simulink model "TST_MeUn_VD"  (R2016b)
settings: Solver=FixedStepDiscrete  StartTime=0.0  StopTime=simTime  FixedStep=sampleTime  RelTol=1e-3
values from neighbouring files (symbols this model uses):
  testCase = 1    [initTST_MeUn_VD_001.m]
libraries: simulink x9, UnitTest_Lib x7
settings Model: Creator=zhengjinyan  LastModifiedBy=zhengjinyan
settings DebuggingCC: SignalRangeChecking=error

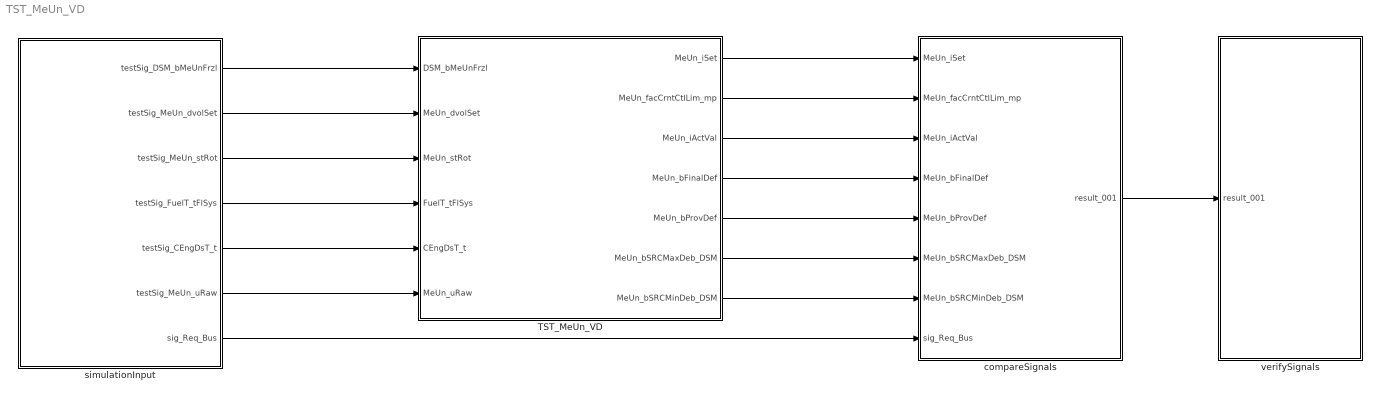
== system TST_MeUn_VD ==
  TST_MeUn_VD : Subsystem
  compareSignals : Subsystem
  simulationInput : Subsystem
  verifySignals : Subsystem
  wires:
  simulationInput/1(testSig_DSM_bMeUnFrzl) -> TST_MeUn_VD/1(DSM_bMeUnFrzl)
  simulationInput/2(testSig_MeUn_dvolSet) -> TST_MeUn_VD/2(MeUn_dvolSet)
  simulationInput/3(testSig_MeUn_stRot) -> TST_MeUn_VD/3(MeUn_stRot)
  simulationInput/4(testSig_FuelT_tFlSys) -> TST_MeUn_VD/4(FuelT_tFlSys)
  simulationInput/5(testSig_CEngDsT_t) -> TST_MeUn_VD/5(CEngDsT_t)
  simulationInput/6(testSig_MeUn_uRaw) -> TST_MeUn_VD/6(MeUn_uRaw)
  TST_MeUn_VD/1(MeUn_iSet) -> compareSignals/1(MeUn_iSet)
  TST_MeUn_VD/2(MeUn_facCrntCtlLim_mp) -> compareSignals/2(MeUn_facCrntCtlLim_mp)
  TST_MeUn_VD/3(MeUn_iActVal) -> compareSignals/3(MeUn_iActVal)
  TST_MeUn_VD/4(MeUn_bFinalDef) -> compareSignals/4(MeUn_bFinalDef)
  TST_MeUn_VD/5(MeUn_bProvDef) -> compareSignals/5(MeUn_bProvDef)
  TST_MeUn_VD/6(MeUn_bSRCMaxDeb_DSM) -> compareSignals/6(MeUn_bSRCMaxDeb_DSM)
  TST_MeUn_VD/7(MeUn_bSRCMinDeb_DSM) -> compareSignals/7(MeUn_bSRCMinDeb_DSM)
  simulationInput/7(sig_Req_Bus) -> compareSignals/8(sig_Req_Bus)
  compareSignals/1(result_001) -> verifySignals/1(result_001)

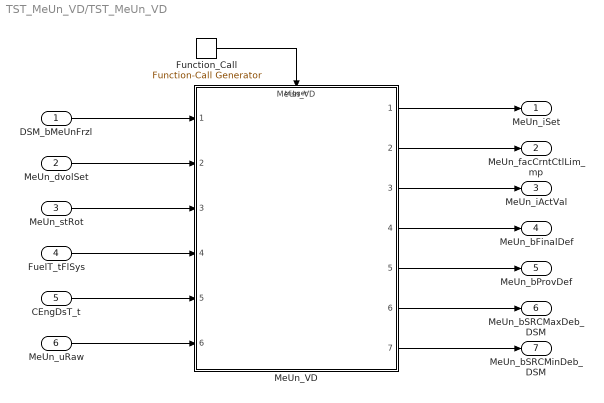
== system TST_MeUn_VD/TST_MeUn_VD ==
  DSM_bMeUnFrzl : Inport
  MeUn_dvolSet : Inport  Port=2
  MeUn_stRot : Inport  Port=3
  FuelT_tFlSys : Inport  Port=4
  CEngDsT_t : Inport  Port=5
  MeUn_uRaw : Inport  Port=6
  Function_Call : simulink/Ports & Subsystems/Function-Call Generator  sample_time=sampleTime  numberOfIterations=1
  MeUn_VD : ModelReference  ModelNameDialog=MeUn_VD  SimulationMode=Normal  ModelReferenceVersion=1.27  TriggerPortName=function  TriggerPortTriggerType=function-call  TriggerPortStatesWhenEnabling=held
  MeUn_iSet : Outport
  MeUn_facCrntCtlLim_mp : Outport  Port=2
  MeUn_iActVal : Outport  Port=3
  MeUn_bFinalDef : Outport  Port=4
  MeUn_bProvDef : Outport  Port=5
  MeUn_bSRCMaxDeb_DSM : Outport  Port=6
  MeUn_bSRCMinDeb_DSM : Outport  Port=7
  wires:
  Function_Call/1 -> MeUn_VD/Trigger
  DSM_bMeUnFrzl/1 -> MeUn_VD/1
  MeUn_dvolSet/1 -> MeUn_VD/2
  MeUn_stRot/1 -> MeUn_VD/3
  FuelT_tFlSys/1 -> MeUn_VD/4
  CEngDsT_t/1 -> MeUn_VD/5
  MeUn_uRaw/1 -> MeUn_VD/6
  MeUn_VD/1 -> MeUn_iSet/1
  MeUn_VD/2 -> MeUn_facCrntCtlLim_mp/1
  MeUn_VD/3 -> MeUn_iActVal/1
  MeUn_VD/4 -> MeUn_bFinalDef/1
  MeUn_VD/5 -> MeUn_bProvDef/1
  MeUn_VD/6 -> MeUn_bSRCMaxDeb_DSM/1
  MeUn_VD/7 -> MeUn_bSRCMinDeb_DSM/1

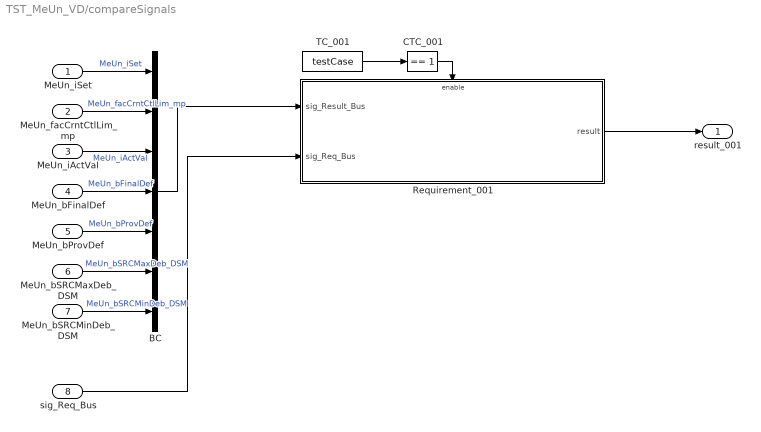
== system TST_MeUn_VD/compareSignals ==
  MeUn_iSet : Inport
  MeUn_facCrntCtlLim_mp : Inport  Port=2
  MeUn_iActVal : Inport  Port=3
  MeUn_bFinalDef : Inport  Port=4
  MeUn_bProvDef : Inport  Port=5
  MeUn_bSRCMaxDeb_DSM : Inport  Port=6
  MeUn_bSRCMinDeb_DSM : Inport  Port=7
  sig_Req_Bus : Inport  Port=8
  BC : BusCreator  Inputs=7
  CTC_001 : simulink/Logic and Bit Operations/Compare To Constant  relop===  const=1  OutDataTypeStr=boolean
  Requirement_001 : Subsystem
  TC_001 : Constant  Value=testCase
  result_001 : Outport
  wires:
  MeUn_iSet/1 -> BC/1  "MeUn_iSet"
  MeUn_facCrntCtlLim_mp/1 -> BC/2  "MeUn_facCrntCtlLim_mp"
  MeUn_iActVal/1 -> BC/3  "MeUn_iActVal"
  MeUn_bFinalDef/1 -> BC/4  "MeUn_bFinalDef"
  MeUn_bProvDef/1 -> BC/5  "MeUn_bProvDef"
  MeUn_bSRCMaxDeb_DSM/1 -> BC/6  "MeUn_bSRCMaxDeb_DSM"
  MeUn_bSRCMinDeb_DSM/1 -> BC/7  "MeUn_bSRCMinDeb_DSM"
  TC_001/1 -> CTC_001/1
  CTC_001/1 -> Requirement_001/Enable
  sig_Req_Bus/1 -> Requirement_001/2(sig_Req_Bus)
  BC/1 -> Requirement_001/1(sig_Result_Bus)
  Requirement_001/1(result) -> result_001/1

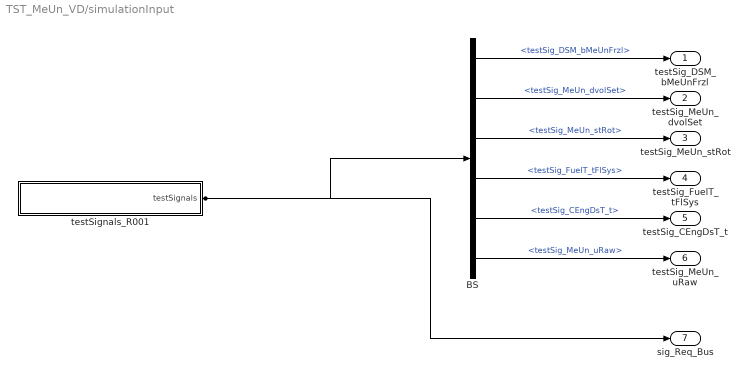
== system TST_MeUn_VD/simulationInput ==
  BS : BusSelector  OutputSignals=testSig_DSM_bMeUnFrzl,testSig_MeUn_dvolSet,testSig_MeUn_stRot,testSig_FuelT_tFlSys,testSig_CEngDsT_t,testSig_MeUn_uRaw
  testSignals_R001 : Subsystem
  testSig_DSM_bMeUnFrzl : Outport
  testSig_MeUn_dvolSet : Outport  Port=2
  testSig_MeUn_stRot : Outport  Port=3
  testSig_FuelT_tFlSys : Outport  Port=4
  testSig_CEngDsT_t : Outport  Port=5
  testSig_MeUn_uRaw : Outport  Port=6
  sig_Req_Bus : Outport  Port=7
  wires:
  BS/1 -> testSig_DSM_bMeUnFrzl/1  "<testSig_DSM_bMeUnFrzl>"
  BS/2 -> testSig_MeUn_dvolSet/1  "<testSig_MeUn_dvolSet>"
  BS/3 -> testSig_MeUn_stRot/1  "<testSig_MeUn_stRot>"
  BS/4 -> testSig_FuelT_tFlSys/1  "<testSig_FuelT_tFlSys>"
  BS/5 -> testSig_CEngDsT_t/1  "<testSig_CEngDsT_t>"
  BS/6 -> testSig_MeUn_uRaw/1  "<testSig_MeUn_uRaw>"
  testSignals_R001/1(testSignals) -> BS/1, sig_Req_Bus/1

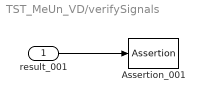
== system TST_MeUn_VD/verifySignals ==
  result_001 : Inport
  Assertion_001 : Assertion  Enabled=off
  wires:
  result_001/1 -> Assertion_001/1

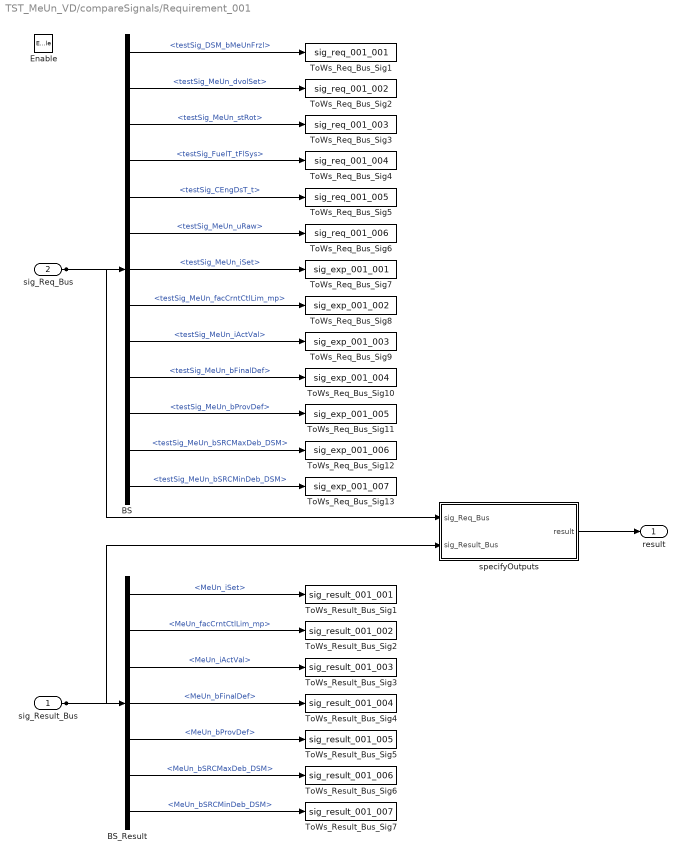
== system TST_MeUn_VD/compareSignals/Requirement_001 ==
  sig_Result_Bus : Inport
  sig_Req_Bus : Inport  Port=2
  Enable : EnablePort
  BS : BusSelector  OutputSignals=testSig_DSM_bMeUnFrzl,testSig_MeUn_dvolSet,testSig_MeUn_stRot,testSig_FuelT_tFlSys,testSig_CEngDsT_t,testSig_MeUn_uRaw,testSig_MeUn_iSet,testSig_MeUn_facCrntCtlLim_mp,testSig_MeUn_iActVal,testSig_MeUn_bFinalDef,testSig_MeUn_bProvDef,testSig_MeUn_bSRCMaxDeb_DSM,testSig_MeUn_bSRCMinDeb_DSM
  BS_Result : BusSelector  OutputSignals=MeUn_iSet,MeUn_facCrntCtlLim_mp,MeUn_iActVal,MeUn_bFinalDef,MeUn_bProvDef,MeUn_bSRCMaxDeb_DSM,MeUn_bSRCMinDeb_DSM
  ToWs_Req_Bus_Sig1 : ToWorkspace  VariableName=sig_req_001_001  SaveFormat=Structure With Time
  ToWs_Req_Bus_Sig10 : ToWorkspace  VariableName=sig_exp_001_004  SaveFormat=Structure With Time
  ToWs_Req_Bus_Sig11 : ToWorkspace  VariableName=sig_exp_001_005  SaveFormat=Structure With Time
  ToWs_Req_Bus_Sig12 : ToWorkspace  VariableName=sig_exp_001_006  SaveFormat=Structure With Time
  ToWs_Req_Bus_Sig13 : ToWorkspace  VariableName=sig_exp_001_007  SaveFormat=Structure With Time
  ToWs_Req_Bus_Sig2 : ToWorkspace  VariableName=sig_req_001_002  SaveFormat=Structure With Time
  ToWs_Req_Bus_Sig3 : ToWorkspace  VariableName=sig_req_001_003  SaveFormat=Structure With Time
  ToWs_Req_Bus_Sig4 : ToWorkspace  VariableName=sig_req_001_004  SaveFormat=Structure With Time
  ToWs_Req_Bus_Sig5 : ToWorkspace  VariableName=sig_req_001_005  SaveFormat=Structure With Time
  ToWs_Req_Bus_Sig6 : ToWorkspace  VariableName=sig_req_001_006  SaveFormat=Structure With Time
  ToWs_Req_Bus_Sig7 : ToWorkspace  VariableName=sig_exp_001_001  SaveFormat=Structure With Time
  ToWs_Req_Bus_Sig8 : ToWorkspace  VariableName=sig_exp_001_002  SaveFormat=Structure With Time
  ToWs_Req_Bus_Sig9 : ToWorkspace  VariableName=sig_exp_001_003  SaveFormat=Structure With Time
  ToWs_Result_Bus_Sig1 : ToWorkspace  VariableName=sig_result_001_001  SaveFormat=Structure With Time
  ToWs_Result_Bus_Sig2 : ToWorkspace  VariableName=sig_result_001_002  SaveFormat=Structure With Time
  ToWs_Result_Bus_Sig3 : ToWorkspace  VariableName=sig_result_001_003  SaveFormat=Structure With Time
  ToWs_Result_Bus_Sig4 : ToWorkspace  VariableName=sig_result_001_004  SaveFormat=Structure With Time
  ToWs_Result_Bus_Sig5 : ToWorkspace  VariableName=sig_result_001_005  SaveFormat=Structure With Time
  ToWs_Result_Bus_Sig6 : ToWorkspace  VariableName=sig_result_001_006  SaveFormat=Structure With Time
  ToWs_Result_Bus_Sig7 : ToWorkspace  VariableName=sig_result_001_007  SaveFormat=Structure With Time
  specifyOutputs : Subsystem
  result : Outport
  wires:
  sig_Req_Bus/1 -> BS/1, specifyOutputs/1(sig_Req_Bus)
  BS/1 -> ToWs_Req_Bus_Sig1/1  "<testSig_DSM_bMeUnFrzl>"
  BS/2 -> ToWs_Req_Bus_Sig2/1  "<testSig_MeUn_dvolSet>"
  BS/3 -> ToWs_Req_Bus_Sig3/1  "<testSig_MeUn_stRot>"
  BS/4 -> ToWs_Req_Bus_Sig4/1  "<testSig_FuelT_tFlSys>"
  BS/5 -> ToWs_Req_Bus_Sig5/1  "<testSig_CEngDsT_t>"
  BS/6 -> ToWs_Req_Bus_Sig6/1  "<testSig_MeUn_uRaw>"
  BS/7 -> ToWs_Req_Bus_Sig7/1  "<testSig_MeUn_iSet>"
  BS/8 -> ToWs_Req_Bus_Sig8/1  "<testSig_MeUn_facCrntCtlLim_mp>"
  BS/9 -> ToWs_Req_Bus_Sig9/1  "<testSig_MeUn_iActVal>"
  BS/10 -> ToWs_Req_Bus_Sig10/1  "<testSig_MeUn_bFinalDef>"
  BS/11 -> ToWs_Req_Bus_Sig11/1  "<testSig_MeUn_bProvDef>"
  BS/12 -> ToWs_Req_Bus_Sig12/1  "<testSig_MeUn_bSRCMaxDeb_DSM>"
  BS/13 -> ToWs_Req_Bus_Sig13/1  "<testSig_MeUn_bSRCMinDeb_DSM>"
  sig_Result_Bus/1 -> BS_Result/1, specifyOutputs/2(sig_Result_Bus)
  BS_Result/1 -> ToWs_Result_Bus_Sig1/1  "<MeUn_iSet>"
  BS_Result/2 -> ToWs_Result_Bus_Sig2/1  "<MeUn_facCrntCtlLim_mp>"
  BS_Result/3 -> ToWs_Result_Bus_Sig3/1  "<MeUn_iActVal>"
  BS_Result/4 -> ToWs_Result_Bus_Sig4/1  "<MeUn_bFinalDef>"
  BS_Result/5 -> ToWs_Result_Bus_Sig5/1  "<MeUn_bProvDef>"
  BS_Result/6 -> ToWs_Result_Bus_Sig6/1  "<MeUn_bSRCMaxDeb_DSM>"
  BS_Result/7 -> ToWs_Result_Bus_Sig7/1  "<MeUn_bSRCMinDeb_DSM>"
  specifyOutputs/1(result) -> result/1

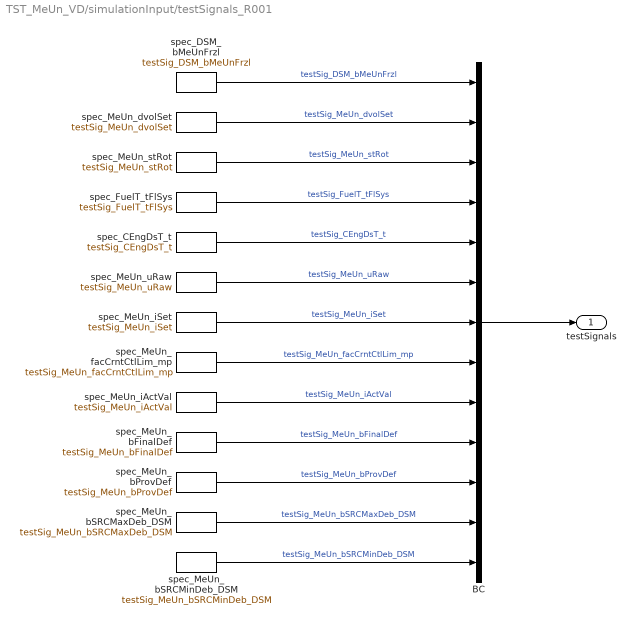
== system TST_MeUn_VD/simulationInput/testSignals_R001 ==
  BC : BusCreator  Inputs=13
  spec_CEngDsT_t : FromWorkspace  VariableName=testSig_CEngDsT_t  Interpolate=off  OutputAfterFinalValue=Holding final value
  spec_DSM_bMeUnFrzl : FromWorkspace  VariableName=testSig_DSM_bMeUnFrzl  Interpolate=off  OutputAfterFinalValue=Holding final value
  spec_FuelT_tFlSys : FromWorkspace  VariableName=testSig_FuelT_tFlSys  Interpolate=off  OutputAfterFinalValue=Holding final value
  spec_MeUn_bFinalDef : FromWorkspace  VariableName=testSig_MeUn_bFinalDef  Interpolate=off  OutputAfterFinalValue=Holding final value
  spec_MeUn_bProvDef : FromWorkspace  VariableName=testSig_MeUn_bProvDef  Interpolate=off  OutputAfterFinalValue=Holding final value
  spec_MeUn_bSRCMaxDeb_DSM : FromWorkspace  VariableName=testSig_MeUn_bSRCMaxDeb_DSM  Interpolate=off  OutputAfterFinalValue=Holding final value
  spec_MeUn_bSRCMinDeb_DSM : FromWorkspace  VariableName=testSig_MeUn_bSRCMinDeb_DSM  Interpolate=off  OutputAfterFinalValue=Holding final value
  spec_MeUn_dvolSet : FromWorkspace  VariableName=testSig_MeUn_dvolSet  Interpolate=off  OutputAfterFinalValue=Holding final value
  spec_MeUn_facCrntCtlLim_mp : FromWorkspace  VariableName=testSig_MeUn_facCrntCtlLim_mp  Interpolate=off  OutputAfterFinalValue=Holding final value
  spec_MeUn_iActVal : FromWorkspace  VariableName=testSig_MeUn_iActVal  Interpolate=off  OutputAfterFinalValue=Holding final value
  spec_MeUn_iSet : FromWorkspace  VariableName=testSig_MeUn_iSet  Interpolate=off  OutputAfterFinalValue=Holding final value
  spec_MeUn_stRot : FromWorkspace  VariableName=testSig_MeUn_stRot  Interpolate=off  OutputAfterFinalValue=Holding final value
  spec_MeUn_uRaw : FromWorkspace  VariableName=testSig_MeUn_uRaw  Interpolate=off  OutputAfterFinalValue=Holding final value
  testSignals : Outport
  wires:
  BC/1 -> testSignals/1
  spec_DSM_bMeUnFrzl/1 -> BC/1  "testSig_DSM_bMeUnFrzl"
  spec_MeUn_dvolSet/1 -> BC/2  "testSig_MeUn_dvolSet"
  spec_MeUn_stRot/1 -> BC/3  "testSig_MeUn_stRot"
  spec_FuelT_tFlSys/1 -> BC/4  "testSig_FuelT_tFlSys"
  spec_CEngDsT_t/1 -> BC/5  "testSig_CEngDsT_t"
  spec_MeUn_uRaw/1 -> BC/6  "testSig_MeUn_uRaw"
  spec_MeUn_iSet/1 -> BC/7  "testSig_MeUn_iSet"
  spec_MeUn_facCrntCtlLim_mp/1 -> BC/8  "testSig_MeUn_facCrntCtlLim_mp"
  spec_MeUn_iActVal/1 -> BC/9  "testSig_MeUn_iActVal"
  spec_MeUn_bFinalDef/1 -> BC/10  "testSig_MeUn_bFinalDef"
  spec_MeUn_bProvDef/1 -> BC/11  "testSig_MeUn_bProvDef"
  spec_MeUn_bSRCMaxDeb_DSM/1 -> BC/12  "testSig_MeUn_bSRCMaxDeb_DSM"
  spec_MeUn_bSRCMinDeb_DSM/1 -> BC/13  "testSig_MeUn_bSRCMinDeb_DSM"

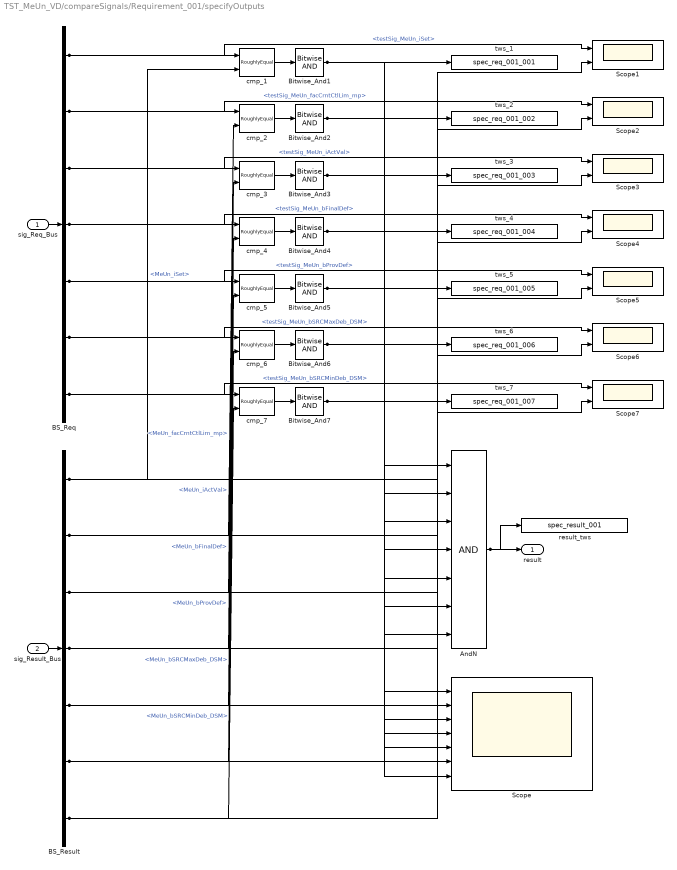
== system TST_MeUn_VD/compareSignals/Requirement_001/specifyOutputs ==
  sig_Req_Bus : Inport
  sig_Result_Bus : Inport  Port=2
  AndN : Logic  Inputs=7
  BS_Req : BusSelector  OutputSignals=testSig_MeUn_iSet,testSig_MeUn_facCrntCtlLim_mp,testSig_MeUn_iActVal,testSig_MeUn_bFinalDef,testSig_MeUn_bProvDef,testSig_MeUn_bSRCMaxDeb_DSM,testSig_MeUn_bSRCMinDeb_DSM
  BS_Result : BusSelector  OutputSignals=MeUn_iSet,MeUn_facCrntCtlLim_mp,MeUn_iActVal,MeUn_bFinalDef,MeUn_bProvDef,MeUn_bSRCMaxDeb_DSM,MeUn_bSRCMinDeb_DSM
  Bitwise_And{1..7} (7 alike) : simulink/Logic and Bit Operations/Bitwise Operator  logicop=AND  UseBitMask=off  BitMask=bin2dec('11011001')  BitMaskRealWorld=Stored Integer
  Scope : Scope  NumInputPorts=7
  Scope{1..7} (7 alike) : Scope  NumInputPorts=2
  cmp_{1..7} (7 alike) : UnitTest_Lib/RoughlyEqual  slope=0.1
  result_tws : ToWorkspace  VariableName=spec_result_001
  tws_1 : ToWorkspace  VariableName=spec_req_001_001
  tws_2 : ToWorkspace  VariableName=spec_req_001_002
  tws_3 : ToWorkspace  VariableName=spec_req_001_003
  tws_4 : ToWorkspace  VariableName=spec_req_001_004
  tws_5 : ToWorkspace  VariableName=spec_req_001_005
  tws_6 : ToWorkspace  VariableName=spec_req_001_006
  tws_7 : ToWorkspace  VariableName=spec_req_001_007
  result : Outport
  wires:
  sig_Req_Bus/1 -> BS_Req/1
  sig_Result_Bus/1 -> BS_Result/1
  AndN/1 -> result/1, result_tws/1
  BS_Req/1 -> cmp_1/1, Scope1/1  "<testSig_MeUn_iSet>"
  BS_Result/1 -> cmp_1/2, Scope1/2  "<MeUn_iSet>"
  cmp_1/1 -> Bitwise_And1/1
  Bitwise_And1/1 -> tws_1/1, AndN/1, Scope/1
  BS_Req/2 -> cmp_2/1, Scope2/1  "<testSig_MeUn_facCrntCtlLim_mp>"
  BS_Result/2 -> cmp_2/2, Scope2/2  "<MeUn_facCrntCtlLim_mp>"
  cmp_2/1 -> Bitwise_And2/1
  Bitwise_And2/1 -> tws_2/1, AndN/2, Scope/2
  BS_Req/3 -> cmp_3/1, Scope3/1  "<testSig_MeUn_iActVal>"
  BS_Result/3 -> cmp_3/2, Scope3/2  "<MeUn_iActVal>"
  cmp_3/1 -> Bitwise_And3/1
  Bitwise_And3/1 -> tws_3/1, AndN/3, Scope/3
  BS_Req/4 -> cmp_4/1, Scope4/1  "<testSig_MeUn_bFinalDef>"
  BS_Result/4 -> cmp_4/2, Scope4/2  "<MeUn_bFinalDef>"
  cmp_4/1 -> Bitwise_And4/1
  Bitwise_And4/1 -> tws_4/1, AndN/4, Scope/4
  BS_Req/5 -> cmp_5/1, Scope5/1  "<testSig_MeUn_bProvDef>"
  BS_Result/5 -> cmp_5/2, Scope5/2  "<MeUn_bProvDef>"
  cmp_5/1 -> Bitwise_And5/1
  Bitwise_And5/1 -> tws_5/1, AndN/5, Scope/5
  BS_Req/6 -> cmp_6/1, Scope6/1  "<testSig_MeUn_bSRCMaxDeb_DSM>"
  BS_Result/6 -> cmp_6/2, Scope6/2  "<MeUn_bSRCMaxDeb_DSM>"
  cmp_6/1 -> Bitwise_And6/1
  Bitwise_And6/1 -> tws_6/1, AndN/6, Scope/6
  BS_Req/7 -> cmp_7/1, Scope7/1  "<testSig_MeUn_bSRCMinDeb_DSM>"
  BS_Result/7 -> cmp_7/2, Scope7/2  "<MeUn_bSRCMinDeb_DSM>"
  cmp_7/1 -> Bitwise_And7/1
  Bitwise_And7/1 -> tws_7/1, AndN/7, Scope/7
